simulink library "SimscapeCustomComponents_lib"  (R2025b)
settings: Solver=VariableStepAuto  StartTime=0.0  StopTime=10.0  RelTol=1e-3
undefined symbols (not defined in the file or in its folder): base, baseVdc, capacity, DiscIntNeverNeededParam, ee_sli_rtmsupport, filterInductance, freqeuncy, frequency, gcbh, gflInverter, gfmInverter, iMaxPU, Inertia, initialSOC, plantRating, solar, Ts, ups, Vac, windSystem, windTurbine
libraries: fl_lib x397, nesl_utility x171, eeGeneralControl x85, ee_lib x82, simulink x72, datacenter_lib x68, eeTransforms x38, slpidlib x24, buildingEnergy_lib x20, SimscapeFluids_lib x17, eeSinusoidalMeasurementV2 x8, eePwmGenerator x8
(part 1 of 24)
settings Model: Creator=skota  LastModifiedBy=skota

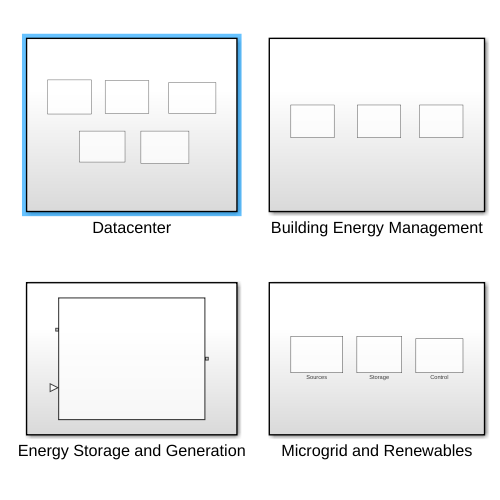
[thumbnail: Simulink's stored preview of the top-level diagram]
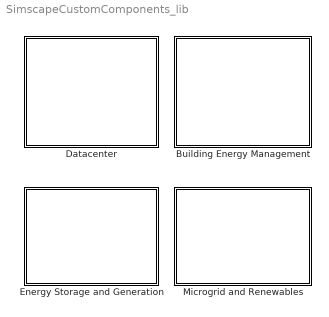
== system SimscapeCustomComponents_lib ==
  Building Energy Management : Subsystem
  Datacenter : Subsystem
  Energy Storage and Generation : Subsystem
  Microgrid and Renewables : Subsystem

== system SimscapeCustomComponents_lib/Building Energy Management ==
  Building : Subsystem
  Environment : Subsystem
  HVAC : Subsystem

== system SimscapeCustomComponents_lib/Datacenter ==
  Assemblies : Subsystem
  CDU : Subsystem
  Facilities : Subsystem
  PDU : Subsystem
  Utilities : Subsystem

== system SimscapeCustomComponents_lib/Energy Storage and Generation ==
  Vanadium Redox Flow Battery : energyStorage_lib/Vanadium Redox Flow Battery  flowrateLUT=[5, 10, 20, 40, 80] lpm  thermalManagement=vanadiumRedoxFlowThermalModel.disabled  temperatureLUT=[293, 300, 313] K  initialTsys=280 K  SOC=0.99  electrolyteDen=1000 kg/m^3  electrolyteCp=800 J/(K*kg)  electrolyteKinVis=3.9e-6 m^2/s  crossDiffModel=vanadiumRedoxFlowChemistry.disabled  thMemb=1e-3 m  diffCoeff2=4.31e-12 m^2/s  diffCoeff3=1.92e-12 m^2/s  diffCoeff4=6.53e-12 m^2/s  diffCoeff5=3.78e-12 m^2/s  activationE=17341 W*s/mol  electrolyteK=1 1/(Ohm*m)  minStateOfCharge=1e-4  maxStateOfCharge=0.9999  msgWarn=simscape.enum.assert.action.none  molar=2 mol/l  V0=1.3 V  LUTdischgR0=0.1 * ones(1, 5) Ohm  LUTdischgRes=0.1 * ones(1, 5) Ohm  LUTdischgTau=10 * ones(1, 5) s  LUTchgR0=0.1 * ones(1, 5) Ohm  LUTchgRes=0.1 * ones(1, 5) Ohm  LUTchgTau=10 * ones(1, 5) s  stackLen=0.15 m  stackWid=0.30 m  stackHgt=0.30 m  stackMassCp=324000 J/K  stackPrDropLUT=[100, 110, 120, 130, 140] Pa  pipeLength=1 m  pipeDia=1e-2 m  pipeArea=0.01 m^2  pipeRoughness=15e-6 m  Nc=20  Ns=10  Np=2  seriesFlowMalDistr=ones(1, 10)  shuntResModel=vanadiumRedoxFlowShuntCurrModel.disabled  shuntRes=1000 Ohm  containerVolume=0.5 m^3  containerArea=10 m^2  containerThermalmass=90000 J/K  nFans=5  fanCapacity=80 m^3/hr  extHTC=20 W/(K*m^2)  F=96485 C/mol  R=8.314 J/(K*mol)  Cmin=0 mol/m^3  openSw=1e-8 1/Ohm  flUnit=1 / 60000 m^3/(lpm*s)  containerAirCp=700 J/(K*kg)  containerAirDen=1.2 kg/m^3  ReLaminar=2000  ReTurbulent=4000  darcyFriction=64  vSwitchOpen_specify=off  vSwitchOpen_priority=None  vSwitchOpen=0 V  vSwitchOpen_nominal_specify=off  vSwitchOpen_nominal_value=1  vSwitchOpen_nominal_unit=V  portH_specify=off  portH_priority=None  portH=0 W  portH_nominal_specify=off  portH_nominal_value=1  portH_nominal_unit=W  tankNegT_specify=off  tankNegT_priority=High  tankNegT=298 K  tankNegT_nominal_specify=off  tankNegT_nominal_value=1  tankNegT_nominal_unit=K  tankPosT_specify=off  tankPosT_priority=High  tankPosT=298 K  tankPosT_nominal_specify=off  tankPosT_nominal_value=1  tankPosT_nominal_unit=K  i_specify=off  i_priority=None  i=0 A  i_nominal_specify=off  i_nominal_value=1  i_nominal_unit=A  is_specify=off  is_priority=None  is=0 A  is_nominal_specify=off  is_nominal_value=1  is_nominal_unit=A  systemPrDrop_specify=off  systemPrDrop_priority=None  systemPrDrop=0 Pa  systemPrDrop_nominal_specify=off  systemPrDrop_nominal_value=1  systemPrDrop_nominal_unit=Pa  shuntCurrPercent_specify=off  shuntCurrPercent_priority=None  shuntCurrPercent=0  shuntCurrPercent_nominal_specify=off  shuntCurrPercent_nominal_value=1  shuntCurrPercent_nominal_unit=1
      settings: InternalSimscapePortConfiguration="{\"Bottom\":[],\"Left\":[{\"id\":\"p\",\"label\":\"+\",\"type\":\"foundation.electrical.electrical\"},{\"id\":\"flow\",\"label\":\"lpm\",\"type\":\"input\"}],\"Right\":[{\"id\":\"n\",\"label\":\"-\",\"type\":\"foundation.electrical.electrical\"}],\"Top\":[]}"

== system SimscapeCustomComponents_lib/Microgrid and Renewables ==
  Control : Subsystem
  Sources : Subsystem
  Storage : Subsystem

== system SimscapeCustomComponents_lib/Building Energy Management/Building ==
  Room Volume : buildingEnergy_lib/Room Volume  N1=1  N2=1  iniT=300 K  length=5 m  width=3 m  height=2.5 m
      settings: InternalSimscapePortConfiguration="{\"Bottom\":[],\"Left\":[{\"id\":\"S\",\"label\":\"S\",\"type\":\"input\"}],\"Right\":[{\"id\":\"T\",\"label\":\"T\",\"type\":\"output\"}],\"Top\":[{\"id\":\"M1\",\"label\":\"M1\",\"type\":\"foundation.thermal.thermal\"},{\"id\":\"M2\",\"label\":\"M2\",\"type\":\"foundation.thermal.thermal\"}]}"
  Room Volume (HVAC) : buildingEnergy_lib/Room Volume (HVAC)  Hnum=1  length=5 m  width=3 m  height=2.5 m  airInletCrossSection=0.01 m^2  airOutletCrossSection=0.01 m^2  perPersonQ=0 W  breathT=0 K  perPersonCO2=0 g/s  perPersonMoisture=0 g/s  relHumidity=1  tauCondensation=0.001 s  entrainedFrac=1  traceGasMassFrac=0  pressureAirVol=0.101325 MPa  temperatureAirVol=293 K  relHumidityAirVol=0  mfWaterDroplets=0
      settings: InternalSimscapePortConfiguration="{\"Bottom\":[],\"Left\":[{\"id\":\"S\",\"label\":\"S\",\"type\":\"input\"},{\"id\":\"N\",\"label\":\"N\",\"type\":\"input\"},{\"id\":\"A\",\"label\":\"A\",\"type\":\"foundation.moist_air.moist_air\"}],\"Right\":[{\"id\":\"T\",\"label\":\"T\",\"type\":\"output\"},{\"id\":\"B\",\"label\":\"B\",\"type\":\"foundation.moist_air.moist_air\"}],\"Top\":[{\"id\":\"H\",\"label\":\"M\",\"type\":\"foundation.thermal.thermal\"}]}"
  Room with Air Volume : Subsystem  mask{roomWid=3, roomHgt=2.5, roomLen=5, htc=10, iniT=300, indxS=1}
      mask prompts: roomWid "Room Width (m)"; roomHgt "Room Height (m)"; roomLen "Room Length (m)"; htc "Heat Transfer Coefficient (W/K*m^2)"; iniT "Initial Temperature (K)"; indxS "Heat source vector index"
      settings: PortSchema="{\"entries\":[{\"content\":{\"sides\":[{\"content\":{\"connectorIds\":[\"LConn1\",\"LConn2\"]},\"type\":\"ConnectorPlacement.EquallySpacedRectSide\",\"uuid\":\"8440f6ae-3089-4f14-af97-f7a7d9c670fb\"},{\"content\":{\"connectorIds\":[\"RConn1\",\"RConn2\"],\"side\":\"RIGHT\"},\"type\":\"ConnectorPlacement.EquallySpacedRectSide\",\"uuid\":\"df84a625-bd6d-46a4-b71c-d411d28f8df6\"},{\"content\":{\"connectorIds\":[\"LConn3\",\"LConn4\"],\"side\":\"TOP\"},\"type\":\"ConnectorPlacement.EquallySpacedRectSide\",\"uuid\":\"90f16a0a-d00c-4f13-8e79-f2f23ea8b565\"},{\"content\":{\"connectorIds\":[\"RConn3\",\"RConn4\"],\"side\":\"BOTTOM\"},\"type\":\"ConnectorPlacement.EquallySpacedRectSide\",\"uuid\":\"4eb9d9d9-e9b4-43a3-a1e1-726815f3b9ff\"}]},\"type\":\"ConnectorPlacement.EquallySpacedConnector\",\"uuid\":\"51dc529f-94b8-407e-b287-301b2c0c8383\"}],\"packageUris\":[\"http://schema.mathworks.com/mf0/Connector/R2020b\"],\"version\":\"1.0\"}"
      mask Help: web("DocumentationCompositeRoom.html")
      mask DialogControl DescGroupVar Prompt: Description
      mask DialogControl DescTextVar Prompt: Room model with air volume.
      mask DialogControl ParameterGroupRoom Prompt: Room Dimensions
      mask DialogControl ParameterGroupHT Prompt: Heat Transfer
      mask Display: image("roomWithAirVolume.png");
  Room with Radiator : Subsystem  mask{pipeRoughnessR=1e-6, pipeLenR=10, pipeCrossSectionalAreaR=1.75e-4, pipeHydrDiaR=1.5e-2, roomWid=3, roomHgt=2.5, roomLen=5, htc=10, iniT=300, indxS=1, indxV=1}
      mask prompts: pipeRoughnessR "Pipe roughness (m)"; pipeLenR "Pipe length (m)"; pipeCrossSectionalAreaR "Pipe cross-sectional area (m^2)"; pipeHydrDiaR "Pipe hydraulic diameter (m)"; roomWid "Room Width (m)"; roomHgt "Room Height (m)"; roomLen "Room Length (m)"; htc "Heat Transfer Coefficient (W/K*m^2)"; iniT "Initial Temperature (K)"; indxS "Heat source vector index"; indxV "Valve operation vector index"
      settings: PortSchema="{\"entries\":[{\"content\":{\"sides\":[{\"content\":{\"connectorIds\":[\"LConn1\",\"LConn2\",\"LConn3\",\"LConn4\"]},\"type\":\"ConnectorPlacement.EquallySpacedRectSide\",\"uuid\":\"8440f6ae-3089-4f14-af97-f7a7d9c670fb\"},{\"content\":{\"connectorIds\":[\"RConn1\",\"RConn2\",\"RConn3\"],\"side\":\"RIGHT\"},\"type\":\"ConnectorPlacement.EquallySpacedRectSide\",\"uuid\":\"df84a625-bd6d-46a4-b71c-d411d28f8df6\"},{\"content\":{\"connectorIds\":[\"LConn5\",\"LConn6\"],\"side\":\"TOP\"},\"type\":\"ConnectorPlacement.EquallySpacedRectSide\",\"uuid\":\"90f16a0a-d00c-4f13-8e79-f2f23ea8b565\"},{\"content\":{\"connectorIds\":[\"RConn4\",\"RConn5\"],\"side\":\"BOTTOM\"},\"type\":\"ConnectorPlacement.EquallySpacedRectSide\",\"uuid\":\"4eb9d9d9-e9b4-43a3-a1e1-726815f3b9ff\"}]},\"type\":\"ConnectorPlacement.EquallySpacedConnector\",\"uuid\":\"51dc529f-94b8-407e-b287-301b2c0c8383\"}],\"packageUris\":[\"http://schema.mathworks.com/mf0/Connector/R2020b\"],\"version\":\"1.0\"}"
      mask Help: web("DocumentationCompositeRoomRadiator.html")
      mask DialogControl DescGroupVar Prompt: Description
      mask DialogControl DescTextVar Prompt: Room model with radiator for thermal comfort.
      mask DialogControl ParameterGroupRadiator Prompt: Radiator
      mask DialogControl ParameterGroupRoom Prompt: Room Dimensions
      mask DialogControl ParameterGroupHT Prompt: Heat Transfer
      mask Display: image("roomWithRadiator.png");
  Room with Under-floor Piping : Subsystem  mask{pipeRoughnessUFP=1e-6, pipeLenUFP=50, pipeCrossSectionalAreaUFP=1.75e-4, pipeHydrDiaUFP=1.5e-2, thermalResFloor=100, roomWid=3, roomHgt=2.5, roomLen=5, htc=10, iniT=300, indxS=1, indxV=1}
      mask prompts: pipeRoughnessUFP "Pipe roughness (m)"; pipeLenUFP "Pipe length (m)"; pipeCrossSectionalAreaUFP "Pipe cross-sectional area (m^2)"; pipeHydrDiaUFP "Pipe hydraulic diameter (m)"; thermalResFloor "Thermal resistance to floor (K/W)"; roomWid "Room Width (m)"; roomHgt "Room Height (m)"; roomLen "Room Length (m)"; htc "Heat Transfer Coefficient (W/K*m^2)"; iniT "Initial Temperature (K)"; indxS "Heat source vector index"; indxV "Valve operation vector index"
      settings: PortSchema="{\"entries\":[{\"content\":{\"sides\":[{\"content\":{\"connectorIds\":[\"LConn1\",\"LConn2\",\"LConn3\",\"LConn4\"]},\"type\":\"ConnectorPlacement.EquallySpacedRectSide\",\"uuid\":\"8440f6ae-3089-4f14-af97-f7a7d9c670fb\"},{\"content\":{\"connectorIds\":[\"RConn1\",\"RConn2\",\"RConn3\"],\"side\":\"RIGHT\"},\"type\":\"ConnectorPlacement.EquallySpacedRectSide\",\"uuid\":\"df84a625-bd6d-46a4-b71c-d411d28f8df6\"},{\"content\":{\"connectorIds\":[\"LConn5\",\"LConn6\"],\"side\":\"TOP\"},\"type\":\"ConnectorPlacement.EquallySpacedRectSide\",\"uuid\":\"90f16a0a-d00c-4f13-8e79-f2f23ea8b565\"},{\"content\":{\"connectorIds\":[\"RConn4\",\"RConn5\"],\"side\":\"BOTTOM\"},\"type\":\"ConnectorPlacement.EquallySpacedRectSide\",\"uuid\":\"4eb9d9d9-e9b4-43a3-a1e1-726815f3b9ff\"}]},\"type\":\"ConnectorPlacement.EquallySpacedConnector\",\"uuid\":\"51dc529f-94b8-407e-b287-301b2c0c8383\"}],\"packageUris\":[\"http://schema.mathworks.com/mf0/Connector/R2020b\"],\"version\":\"1.0\"}"
      mask Help: web("DocumentationCompositeRoomUFP.html")
      mask DialogControl DescGroupVar Prompt: Description
      mask DialogControl DescTextVar Prompt: Room model with under-floor piping for thermal comfort.
      mask DialogControl ParameterGroupUFP Prompt: Under Floor Piping
      mask DialogControl ParameterGroupRoom Prompt: Room Dimensions
      mask DialogControl ParameterGroupHT Prompt: Heat Transfer
      mask Display: image("roomWithUFP.png");
  "Room, Radiator, and Under-floor Piping" : Subsystem  mask{pipeRoughnessR=1e-6, pipeLenR=10, pipeCrossSectionalAreaR=1.75e-4, pipeHydrDiaR=1.5e-2, pipeRoughnessUFP=1e-6, pipeLenUFP=50, pipeCrossSectionalAreaUFP=1.75e-4, pipeHydrDiaUFP=1.5e-2, thermalResFloor=100, roomWid=3, roomHgt=2.5, roomLen=5, htc=10, iniT=300, indxS=1, indxV=1}
      mask prompts: pipeRoughnessR "Pipe roughness (m)"; pipeLenR "Pipe length (m)"; pipeCrossSectionalAreaR "Pipe cross-sectional area (m^2)"; pipeHydrDiaR "Pipe hydraulic diameter (m)"; pipeRoughnessUFP "Pipe roughness (m)"; pipeLenUFP "Pipe length (m)"; pipeCrossSectionalAreaUFP "Pipe cross-sectional area (m^2)"; pipeHydrDiaUFP "Pipe hydraulic diameter (m)"; thermalResFloor "Thermal resistance to floor (K/W)"; roomWid "Room Width (m)"; roomHgt "Room Height (m)"; roomLen "Room Length (m)"; htc "Heat Transfer Coefficient (W/K*m^2)"; iniT "Initial Temperature (K)"; indxS "Heat source vector index"; indxV "Valve operation vector index"
      settings: PortSchema="{\"entries\":[{\"content\":{\"sides\":[{\"content\":{\"connectorIds\":[\"LConn1\",\"LConn2\",\"LConn3\",\"LConn4\"]},\"type\":\"ConnectorPlacement.EquallySpacedRectSide\",\"uuid\":\"8440f6ae-3089-4f14-af97-f7a7d9c670fb\"},{\"content\":{\"connectorIds\":[\"RConn1\",\"RConn2\",\"RConn3\"],\"side\":\"RIGHT\"},\"type\":\"ConnectorPlacement.EquallySpacedRectSide\",\"uuid\":\"df84a625-bd6d-46a4-b71c-d411d28f8df6\"},{\"content\":{\"connectorIds\":[\"LConn5\",\"LConn6\"],\"side\":\"TOP\"},\"type\":\"ConnectorPlacement.EquallySpacedRectSide\",\"uuid\":\"90f16a0a-d00c-4f13-8e79-f2f23ea8b565\"},{\"content\":{\"connectorIds\":[\"RConn4\",\"RConn5\"],\"side\":\"BOTTOM\"},\"type\":\"ConnectorPlacement.EquallySpacedRectSide\",\"uuid\":\"4eb9d9d9-e9b4-43a3-a1e1-726815f3b9ff\"}]},\"type\":\"ConnectorPlacement.EquallySpacedConnector\",\"uuid\":\"51dc529f-94b8-407e-b287-301b2c0c8383\"}],\"packageUris\":[\"http://schema.mathworks.com/mf0/Connector/R2020b\"],\"version\":\"1.0\"}"
      mask Help: web("DocumentationCompositeRoomRadiatorUFP.html")
      mask DialogControl DescGroupVar Prompt: Description
      mask DialogControl DescTextVar Prompt: Room model with radiator and under-floor piping for thermal comfort.
      mask DialogControl ParameterGroupRadiator Prompt: Radiator
      mask DialogControl ParameterGroupUFP Prompt: Under Floor Piping
      mask DialogControl ParameterGroupRoom Prompt: Room Dimensions
      mask DialogControl ParameterGroupHT Prompt: Heat Transfer
      mask Display: image("roomWithRadiatorAndUFP.png");
  Wall External : buildingEnergy_lib/Wall External  extWallModel=wallExternalModelOption.wallSolarWinVent  wallLength=5 m  wallHeight=3 m  wallThickness=0.3 m  wallMaterialDen=4000 kg/m^3  wallMaterialCp=1870 J/(K*kg)  wallAbsorptivity=0.5  wallThermalK=2 W/(K*m)  winLength=1 m  winHeight=0.5 m  winThickness=0.007 m  winMaterialDen=2500 kg/m^3  winMaterialCp=787 J/(K*kg)  winAbsorptivity=0.35  winThermalK=1 W/(K*m)  winTransmissivity=0.45  ventLength=0.1 m  ventHeight=0.1 m  extToWallHTC=5 W/(K*m^2)  intToRoomHTC=5 W/(K*m^2)  iniT=300 K  latitude=5  longitude=5  localTime=5  dayLightS=0  surfAngle=90 deg  surfUnitV=[0, -1]  startYear=2025  startMonth=1  startDay=1  startHr=1  numHrsData=24  interp_method=simscape.enum.interpolation.linear  extrap_method=simscape.enum.extrapolation.nearest
      settings: InternalSimscapePortConfiguration="{\"Bottom\":[],\"Left\":[{\"id\":\"R\",\"label\":\"Rad\",\"type\":\"input\"},{\"id\":\"A\",\"label\":\"A\",\"type\":\"foundation.thermal.thermal\"}],\"Right\":[{\"id\":\"B\",\"label\":\"B\",\"type\":\"foundation.thermal.thermal\"}],\"Top\":[]}"
  Wall Selector : buildingEnergy_lib/Wall Selector  optWall=wallModelOption.wallSolarWinVent  wallLength=5 m  wallHeight=3 m  wallThickness=0.3 m  wallMaterialDen=4000 kg/m^3  wallMaterialCp=1870 J/(K*kg)  wallAbsorptivity=0.5  wallThermalK=2 W/(K*m)  winLength=1 m  winHeight=0.5 m  winThickness=0.007 m  winMaterialDen=2500 kg/m^3  winMaterialCp=787 J/(K*kg)  winAbsorptivity=0.35  winThermalK=1 W/(K*m)  winTransmissivity=0.45  ventLength=0.1 m  ventHeight=0.1 m  extToWallHTC=5 W/(K*m^2)  intToRoomHTC=5 W/(K*m^2)  iniT=300 K
      settings: InternalSimscapePortConfiguration="{\"Bottom\":[],\"Left\":[{\"id\":\"S\",\"label\":\"S\",\"type\":\"input\"},{\"id\":\"A\",\"label\":\"A\",\"type\":\"foundation.thermal.thermal\"}],\"Right\":[{\"id\":\"B\",\"label\":\"B\",\"type\":\"foundation.thermal.thermal\"}],\"Top\":[]}"

== system SimscapeCustomComponents_lib/Building Energy Management/Environment ==
  Day Scheduler : buildingEnergy_lib/Day Scheduler  numRoom=30  roomIndex=[1 : 30]  heatSource=ones(30, 24) W  t=1 : 24  oneHr=3600
      settings: InternalSimscapePortConfiguration="{\"Bottom\":[],\"Left\":[],\"Right\":[{\"id\":\"S\",\"label\":\"S\",\"type\":\"output\"}],\"Top\":[]}"
  Solar Radiation (LUT) : buildingEnergy_lib/Solar Radiation (LUT)  latitude=5  longitude=5  localTime=5  dayLightS=0  startYear=2025  startMonth=1  startDay=1  startHr=1  numHrsData=24  cloudData=cloudCoverLibOption.none  cloudCoverVal=zeros(1, 24)  interp_method=simscape.enum.interpolation.linear  extrap_method=simscape.enum.extrapolation.nearest
      settings: InternalSimscapePortConfiguration="{\"Bottom\":[],\"Left\":[],\"Right\":[{\"id\":\"S\",\"label\":\"Rad\",\"type\":\"output\"}],\"Top\":[]}"
  Solar Radiation On Surface : buildingEnergy_lib/Solar Radiation On Surface  latitude=5  longitude=5  localTime=5  dayLightS=0  surfAngle=90 deg  surfUnitV=[0, -1]  startYear=2025  startMonth=1  startDay=1  startHr=1  numHrsData=24  interp_method=simscape.enum.interpolation.linear  extrap_method=simscape.enum.extrapolation.nearest
      settings: InternalSimscapePortConfiguration="{\"Bottom\":[],\"Left\":[{\"id\":\"S\",\"label\":\"Rad\",\"type\":\"input\"}],\"Right\":[{\"id\":\"Sf\",\"label\":\"S\",\"type\":\"output\"}],\"Top\":[]}"
  Temperature Source (LUT) : buildingEnergy_lib/Temperature Source (LUT)  latitude=5  longitude=5  localTime=5  dayLightS=0  startYear=2025  startMonth=1  startDay=1  startHr=1  numDaysData=10  interp_method=simscape.enum.interpolation.linear  extrap_method=simscape.enum.extrapolation.error  avgDayTvec=300 * ones(1, 10) K  pcDayTvar=5  avgNightTvec=300 * ones(1, 10) K  pcNightTvar=5
      settings: InternalSimscapePortConfiguration="{\"Bottom\":[],\"Left\":[],\"Right\":[{\"id\":\"H\",\"label\":\"H\",\"type\":\"foundation.thermal.thermal\"}],\"Top\":[]}"

== system SimscapeCustomComponents_lib/Building Energy Management/HVAC ==
  Air Water Heat Pump : buildingEnergy_lib/Air Water Heat Pump  nominalCapacityA=200 kW  seasonalCOPvalA=3.1  nominalCapacityB=200 kW  seasonalCOPvalB=3.1  nominalCapacityC=200 kW  seasonalCOPvalC=3.1  nominalCapacityD=200 kW  seasonalCOPvalD=3.1  nominalCapacityE=200 kW  seasonalCOPvalE=3.1  nominalCapacityF=200 kW  seasonalCOPvalF=3.1  backupElecHeater=0 kW  wInletOpRangeUpp=330 K  wInletOpRangeLow=278 K  airTemperatureVector=273 + [-2, -2, 7, 7, 35, 35]  waterTemperatureVector=273 + [55, 65, 35, 45, 18, 7]  waterSpHeat=4186 J/(K*kg)  smallPower=1e-3 W  maxCOP_specify=off  maxCOP_priority=None  maxCOP=8  maxCOP_nominal_specify=off  maxCOP_nominal_value=1  maxCOP_nominal_unit=1
      settings: InternalSimscapePortConfiguration="{\"Bottom\":[{\"id\":\"Ta\",\"label\":\"Ta\",\"type\":\"input\"},{\"id\":\"Tw\",\"label\":\"Tw\",\"type\":\"input\"}],\"Left\":[{\"id\":\"Tl\",\"label\":\"Tl\",\"type\":\"input\"},{\"id\":\"Fw\",\"label\":\"Fw\",\"type\":\"input\"},{\"id\":\"Op\",\"label\":\"Op\",\"type\":\"input\"},{\"id\":\"Ep\",\"label\":\"Ep\",\"type\":\"input\"},{\"id\":\"Nd\",\"label\":\"Nd\",\"type\":\"input\"}],\"Right\":[{\"id\":\"calcCap\",\"label\":\"Q\",\"type\":\"output\"},{\"id\":\"calcCOP\",\"label\":\"COP\",\"type\":\"output\"},{\"id\":\"ePower\",\"label\":\"ePow\",\"type\":\"output\"}],\"Top\":[]}"
  Air Water Heat Pump (TL) : Subsystem  mask{heatingCapacityA=10.17, heatingCoPA=4.86, heatingCapacityB=10.12, heatingCoPB=3.7, heatingCapacityC=10.17, heatingCoPC=4.86, heatingCapacityD=10.12, heatingCoPD=3.7, coolingCapacityE=10.55, coolingCoPE=4.13, coolingCapacityF=6.9, coolingCoPF=2.7, elecHeaterPower=0, coilLen=2, coilArea=pi*(5e-2^2)/4, coilDia=5e-2, tankVolume=5, initialT=299.8, waterOpTempMax=330, waterOpTempMin=278, initialP=0.101325, measTimelagWater=60, minWaterFlowRate=1e-3, nomFlowDuringTest=0.5}
      mask prompts: heatingCapacityA "A-2W55, estimated heating capacity (kW)"; heatingCoPA "A-2W55, estimated COP (or SCOP)"; heatingCapacityB "A-2W65, estimated heating capacity (kW)"; heatingCoPB "A-2W65, estimated COP (or SCOP)"; heatingCapacityC "A7W35, estimated heating capacity (kW)"; heatingCoPC "A7W35, estimated COP (or SCOP)"; heatingCapacityD "A7W45, estimated heating capacity (kW)"; heatingCoPD "A7W45, estimated COP (or SCOP)"; coolingCapacityE "A35W18, estimated cooling capacity (kW)"; coolingCoPE "A35W18, estimated COP (or SCOP)"; coolingCapacityF "A35W7, estimated cooling capacity (kW)"; coolingCoPF "A35W7, estimated COP (or SCOP)"; elecHeaterPower "Additional electric heater rating (kW)"; coilLen "Length of coil pipe (m)"; coilArea "Area of coil pipe (m^2)"; coilDia "Diameter of coil pipe (m)"; tankVolume "Heat exchanger internal volume (m^3)"; initialT "Initial Temperature (K)"; waterOpTempMax "Maximum operational water temperature"; waterOpTempMin "Minimum operation water temperature"; initialP "Initial pressure of coil pipe water (MPa)"; measTimelagWater "Temperature sensor delay for water flow (s)"; minWaterFlowRate "Minimum water flowrate (kg/s)"; nomFlowDuringTest "Nominal water flowrate during test (kg/s)"
      mask Help: web("DocumentationAirWaterHeatPumpTL.html")
      mask DialogControl DescGroupVar Prompt: Description
      mask DialogControl DescTextVar Prompt: Heat pump model based on EN14511 test data.
      mask DialogControl Container3 Prompt: EN14511 (Heating) Data
      mask DialogControl Container4 Prompt: EN14511 (Cooling) Data
      mask DialogControl ParameterGroupVar Prompt: Heat Pump Construction
      mask DialogControl Container5 Prompt: Flow and Thermal Specifications
      mask Display: image('AirWaterHeatPumpTL.png');
  Heat Source Control : Subsystem  mask{capacity=12000, num=1, delT=10, tau=1, iniT=280}
      mask prompts: capacity "Heat pump capacity (W)"; num "Number of sources (-)"; delT "Change in water temperature (deg C)"; tau "Measurement time constant (s)"; iniT "Initial water temperature (K)"
      mask Help: web("DocumentationCompositeHeatSourceControl.html")
      mask DialogControl DescGroupVar Prompt: Description
      mask DialogControl DescTextVar Prompt: The block evaluates heating or cooling requirements for a building  based on the measured room temperatures and the specified set point temperature.
      mask DialogControl HeatPump Prompt: Heat Pump
      mask Display: image('HeatSourceControlIcon.png');
  Room Underfloor Piping : buildingEnergy_lib/Room Underfloor Piping  pipeHydrDia=1.5e-2 m  pipeLength=1 m  pipeArea=1.75e-4 m^2  pipeRoughness=1e-6 m  htc=10 W/(K*m^2)  iniTemperature=300 K
      settings: InternalSimscapePortConfiguration="{\"Bottom\":[],\"Left\":[{\"id\":\"TL_V\",\"label\":\"V\",\"type\":\"input\"},{\"id\":\"TL_A\",\"label\":\"A\",\"type\":\"foundation.thermal_liquid.thermal_liquid\"}],\"Right\":[{\"id\":\"M\",\"label\":\"R\",\"type\":\"foundation.thermal.thermal\"},{\"id\":\"TL_B\",\"label\":\"B\",\"type\":\"foundation.thermal_liquid.thermal_liquid\"}],\"Top\":[]}"
  Room Wall Radiator : buildingEnergy_lib/Room Wall Radiator  pipeHydrDia=1.5e-2 m  pipeLength=1 m  pipeArea=1.75e-4 m^2  pipeRoughness=1e-6 m  htc=10 W/(K*m^2)  iniTemperature=300 K
      settings: InternalSimscapePortConfiguration="{\"Bottom\":[],\"Left\":[{\"id\":\"TL_V\",\"label\":\"V\",\"type\":\"input\"},{\"id\":\"TL_A\",\"label\":\"A\",\"type\":\"foundation.thermal_liquid.thermal_liquid\"}],\"Right\":[{\"id\":\"M\",\"label\":\"R\",\"type\":\"foundation.thermal.thermal\"},{\"id\":\"TL_B\",\"label\":\"B\",\"type\":\"foundation.thermal_liquid.thermal_liquid\"}],\"Top\":[]}"

== system SimscapeCustomComponents_lib/Datacenter/Assemblies ==
  Air Cooled PDU Assembly : Subsystem  mask{nAssembly=3, nRacks=4, nTrays=6, nFans=5, flowVec=[0.1 0.2 0.3 0.4 0.5], prDropVec=[50 100 150 220 280], fanEffVec=[0.58, 0.60, 0.61, 0.60, 0.59], trayMass=5, trayCp=2000, trayThermalR=0.1, nGPU=1, gpuTDPperDie=1200, gpuIdlePower=300, gpuHBMpower=80, gpuExponent=1.4, gpuHBMutil=0.7, gpuLeakage=1.5, gpuNominalDieT=350, gpuDieThermalC=50, gpuHeatSinkR=0.15, gpuSurfArea=0.01, gpuAmbientR=0.5, nCPU=1, cpuTDPperSocket=350, cpuIdlePower=80, cpuExponent=1.1, cpuLeakage=1.5, cpuNominalDieT=350, cpuDieThermalC=50, cpuHeatSinkR=0.15, cpuSurfArea=0.01, cpuAmbientR=0.5, initialT=350, htc=10}
      mask prompts: nAssembly "Number of PDU + Fan assemblies (-)"; nRacks "Number of racks per PDU (-)"; nTrays "Number of IT trays per rack (-)"; nFans "Number of fans per assembly (-)"; flowVec "Fan flow rate vector (m^3/s)"; prDropVec "Fan pressure drop vector (Pa)"; fanEffVec "Fan efficiency vector, 0-1 (-)"; trayMass "Tray mass (kg)"; trayCp "Tray specific heat capacity (J/kg*K)"; trayThermalR "Tray to external thermal resistance (K/W)"; nGPU "Number of GPU per tray (-)"; gpuTDPperDie "GPU TDP per die (W)"; gpuIdlePower "GPU idle power (W)"; gpuHBMpower "HBM power per GPU (W)"; gpuExponent "GPU power utilization exponent (-)"; gpuHBMutil "HBM utilization as fraction of compute utilization (-)"; gpuLeakage "Leakage increase per K above nominal temperature (W/K)"; gpuNominalDieT "Nominal die temperature at TDP (K)"; gpuDieThermalC "GPU die thermal capacitance (J/K)"; gpuHeatSinkR "GPU die-heat-sink thermal resistance (K/W)"; gpuSurfArea "Surface area per die for ambient heat transfer (m^2)"; gpuAmbientR "GPU die-ambient thermal resistance (K/W)"; nCPU "Number of CPU per tray (-)"; cpuTDPperSocket "CPU TDP per socket (W)"; cpuIdlePower "CPU idle power per socket (W)"; cpuExponent "CPU power utilization exponent (-)"; cpuLeakage "Leakage increase per K above nominal temperature (W/K)"; cpuNominalDieT "Nominal die temperature at TDP (K)"; cpuDieThermalC "CPU die thermal capacitance (J/K)"; cpuHeatSinkR "CPU die-heat-sink thermal resistance (K/W)"; cpuSurfArea "Surface area per die for ambient heat transfer (m^2)"; cpuAmbientR "CPU die-ambient thermal resistance (K/W)"; initialT "Initial temperature (K)"; htc "Heat transfer coefficient to ambient (W/m^2.K)"
      settings: CopyFcn=set_param(gcbh,'LinkStatus','none');
      mask Help: web("DocumentationAirCooledPDUAssembly.html")
      mask DialogControl Container10 Prompt: PDU Racks
      mask DialogControl getRatingButton Prompt: Get Rating
      mask DialogControl Container11 Prompt: Fans
      mask DialogControl Container9 Prompt: IT Tray
      mask DialogControl Container6 Prompt: GPU
      mask DialogControl Container7 Prompt: CPU
      mask DialogControl Container8 Prompt: Initial Conditions
      mask Display: image('icon_AssemblyAirCooled.png');
  PDU + CDU Assembly (LUT) : Subsystem  mask{nAssembly=3, nRacks=3, nTrays=6, flowrate_vec=[0.3, 0.5, 1.0, 1.3, 1.7, 2, 2.6, 3.3, 3.5, 3.7]/998, capacity_vec=50000*[0.32, 0.35, 0.40, 0.42, 0.43, 0.43, 0.44, 0.45, 0.46, 0.47], numPump=2, effPump_vec=[0.4,0.42,0.45,0.5,0.55,0.6,0.62,0.65,0.65,0.64], prDrop_mat=100000*[0.28,1.11,2.5,4.44,6.94,10,13.61,17.78,22.5,27.78; 5.6,2.22,5,8.88,13.88,20,27.22,35.56,45,55.56]', speed=2, trayMass=5, trayCp=2000, trayThermalR=0.1, nGPU=1, gpuTDPperDie=1200, gpuIdlePower=300, gpuHBMpower=80, gpuExponent=1.4, gpuHBMutil=0.7, gpuLeakage=1.5, gpuNominalDieT=350, gpuDieThermalC=50, gpuHeatSinkR=0.15, gpuSurfArea=0.01, gpuAmbientR=0.5, nCPU=1, cpuTDPperSocket=350, cpuIdlePower=80, cpuExponent=1.1, cpuLeakage=1.5, cpuNominalDieT=350, cpuDieThermalC=50, cpuHeatSinkR=0.15, cpuSurfArea=0.01, cpuAmbientR=0.5, initialT=350, htc=10}
      mask prompts: nAssembly "Number of PDU+CDU assemblies (-)"; nRacks "Number of racks (-)"; nTrays "Number of IT trays per rack (-)"; flowrate_vec "Coolant volumetric flowrate vector (m^3/s)"; capacity_vec "Heat exchanger capacity vector (W)"; numPump "Total number of pumps in each assembly (-)"; effPump_vec "Pump efficiency vector, 0-1 (-)"; prDrop_mat "Pressure drop (Pa)"; speed "Pump speed scaling (-)"; trayMass "Tray mass (kg)"; trayCp "Tray specific heat capacity (J/kg*K)"; trayThermalR "Tray to external thermal resistance (K/W)"; nGPU "Number of GPU per tray (-)"; gpuTDPperDie "GPU TDP per die (W)"; gpuIdlePower "GPU idle power (W)"; gpuHBMpower "HBM power per GPU (W)"; gpuExponent "GPU power utilization exponent (-)"; gpuHBMutil "HBM utilization as fraction of compute utilization (-)"; gpuLeakage "Leakage increase per K above nominal temperature (W/K)"; gpuNominalDieT "Nominal die temperature at TDP (K)"; gpuDieThermalC "GPU die thermal capacitance (J/K)"; gpuHeatSinkR "GPU die-heat-sink thermal resistance (K/W)"; gpuSurfArea "Surface area per die for ambient heat transfer (m^2)"; gpuAmbientR "GPU die-ambient thermal resistance (K/W)"; nCPU "Number of CPU per tray (-)"; cpuTDPperSocket "CPU TDP per socket (W)"; cpuIdlePower "CPU idle power per socket (W)"; cpuExponent "CPU power utilization exponent (-)"; cpuLeakage "Leakage increase per K above nominal temperature (W/K)"; cpuNominalDieT "Nominal die temperature at TDP (K)"; cpuDieThermalC "CPU die thermal capacitance (J/K)"; cpuHeatSinkR "CPU die-heat-sink thermal resistance (K/W)"; cpuSurfArea "Surface area per die for ambient heat transfer (m^2)"; cpuAmbientR "CPU die-ambient thermal resistance (K/W)"; initialT "Initial temperature (K)"; htc "Heat transfer coefficient to ambient (W/m^2.K)"
      settings: CopyFcn=set_param(gcbh,'LinkStatus','none');
      mask Help: web("DocumentationPDUCDUAssemblyLUT.html")
      mask DialogControl Container10 Prompt: PDU Racks
      mask DialogControl getRatingButton Prompt: Get Rating
      mask DialogControl Container11 Prompt: CDU
      mask DialogControl Container9 Prompt: IT Tray
      mask DialogControl Container6 Prompt: GPU
      mask DialogControl Container7 Prompt: CPU
      mask DialogControl Container8 Prompt: Initial Conditions
      mask Display: image('icon_AssemblyLUT.png');
  PDU + CDU Assembly (TL) : Subsystem  mask{nAssembly=3, nTrays=6, nRacks=4, nPumps=1, pumpNominalRPM=3500, pumpCapacityVec=2:2:24, pumpRefHeadVec=[239, 238.5, 232, 230, 222, 216, 208, 196, 186, 170,150,130], pumpRefBrkPowVec=[0.3,0.4,0.45,0.5,0.55,0.6,0.65,0.7,0.75,0.78,0.79,0.798], pumpEff=[20,40,50,60,65,70,75,75,75,73,68,60]/100, speedLimFactor=1, pumpImpellerDiaFactor=1, extFluidMdot=[.3, .5, 1, 1.3, 1.7, 2, 2.6, 3.3], extFluidPrDrop=ones(1,8), extFluidVol=0.01, extFluidPipeArea=0.01, intFluidMdot=[.3, .5, .6, .7, 1, 1.4, 1.9, 2.3], intFluidPrDrop=ones(1,8), intFluidVol=0.01, intFluidPipeArea=0.01, spDissipationTbl=[.324, .3533, .404, .4253, .4333, .4373, .4453, .4533; .3813, .424, .496, .5307, .544, .5547, .5693, .5787; .4267, .4827, .5813, .6173, .6413, .6573, .672, .6827; .4613, .528, .64, .6987, .7267, .7467, .7707, .7853; .5533, .6467, .8227, .928, .9853, 1.0187, 1.0653, 1.0973; .58, .688, .8853, 1.0147, 1.08, 1.124, 1.176, 1.2147; .624, .7467, .992, 1.148, 1.244, 1.304, 1.3773, 1.4267; .656, .7907, 1.0667, 1.26, 1.376, 1.452, 1.548, 1.612], effPipeLen=5, refT=293, refP=0.101325, refDensity=998, trayMass=5, trayCp=2000, trayThermalR=0.1, nGPU=1, gpuTDPperDie=1200, gpuIdlePower=300, gpuHBMpower=80, gpuExponent=1.4, gpuHBMutil=0.7, gpuLeakage=1.5, gpuNominalDieT=350, gpuDieThermalC=50, gpuHeatSinkR=0.15, gpuSurfArea=0.01, gpuAmbientR=0.5, nCPU=1, cpuTDPperSocket=350, cpuIdlePower=80, cpuExponent=1.1, cpuLeakage=1.5, cpuNominalDieT=350, cpuDieThermalC=50, cpuHeatSinkR=0.15, cpuSurfArea=0.01, cpuAmbientR=0.5, initialT=350, initialP=0.101325, htc=10}
      mask prompts: nAssembly "Number of PDU+CDU assemblies (-)"; nTrays "Number of IT trays per rack (-)"; nRacks "Number of racks (-)"; nPumps "Total number of pumps (-)"; pumpNominalRPM "Pump nominal rating (rpm)"; pumpCapacityVec "Reference capacity vector for each pump (m^3/s)"; pumpRefHeadVec "Reference head vector for each pump (m)"; pumpRefBrkPowVec "Reference brake power vector (kW)"; pumpEff "Electrical efficiency vector, 0-1 (-)"; speedLimFactor "Pump speed upper limit factor (-)"; pumpImpellerDiaFactor "Impeller diameter scale factor (-)"; extFluidMdot "External liquid loop mass flow rate vector (kg/s)"; extFluidPrDrop "External liquid loop pressure drop vector (kPa)"; extFluidVol "External liquid volume in heat exchanger (m^3)"; extFluidPipeArea "External liquid loop pipe cross-sectional area (m^2)"; intFluidMdot "Internal liquid loop mass flow rate vector (kg/s)"; intFluidPrDrop "Internal liquid loop pressure drop vector (kPa)"; intFluidVol "Internal liquid volume in heat exchanger (m^3)"; intFluidPipeArea "Internal liquid loop pipe cross-sectional area (m^2)"; spDissipationTbl "Specific dissipation table, SD[mdot_int,mdot_ext] (kW/K)"; effPipeLen "Effective pipe length for rack cooling (m)"; refT "Reference flow temperature (K)"; refP "Reference flow pressure (MPa)"; refDensity "Reference density for internal liquid (kg/m^3)"; trayMass "Tray mass (kg)"; trayCp "Tray specific heat capacity (J/kg*K)"; trayThermalR "Tray to external thermal resistance (K/W)"; nGPU "Number of GPU per tray (-)"; gpuTDPperDie "GPU TDP per die (W)"; gpuIdlePower "GPU idle power (W)"; gpuHBMpower "HBM power per GPU (W)"; gpuExponent "GPU power utilization exponent (-)"; gpuHBMutil "HBM utilization as fraction of compute utilization (-)"; gpuLeakage "Leakage increase per K above nominal temperature (W/K)"; gpuNominalDieT "Nominal die temperature at TDP (K)"; gpuDieThermalC "GPU die thermal capacitance (J/K)"; gpuHeatSinkR "GPU die-heat-sink thermal resistance (K/W)"; gpuSurfArea "Surface area per die for ambient heat transfer (m^2)"; gpuAmbientR "GPU die-ambient thermal resistance (K/W)"; nCPU "Number of CPU per tray (-)"; cpuTDPperSocket "CPU TDP per socket (W)"; cpuIdlePower "CPU idle power per socket (W)"; cpuExponent "CPU power utilization exponent (-)"; cpuLeakage "Leakage increase per K above nominal temperature (W/K)"; cpuNominalDieT "Nominal die temperature at TDP (K)"; cpuDieThermalC "CPU die thermal capacitance (J/K)"; cpuHeatSinkR "CPU die-heat-sink thermal resistance (K/W)"; cpuSurfArea "Surface area per die for ambient heat transfer (m^2)"; cpuAmbientR "CPU die-ambient thermal resistance (K/W)"; initialT "Initial temperature (K)"; initialP "Initial pressure (MPa)"; htc "Heat transfer coefficient to ambient (W/m^2.K)"
      settings: CopyFcn=set_param(gcbh,'LinkStatus','none');  PortSchema="{\"entries\":[{\"content\":{\"sides\":[{\"content\":{\"connectorIds\":[\"LConn1\",\"LConn2\",\"LConn3\",\"LConn4\",\"LConn5\"]},\"type\":\"ConnectorPlacement.EquallySpacedRectSide\",\"uuid\":\"c3c2deed-cbbd-4247-9ad8-92266cae4888\"},{\"content\":{\"connectorIds\":[\"RConn1\",\"RConn2\",\"RConn3\",\"RConn4\"],\"side\":\"RIGHT\"},\"type\":\"ConnectorPlacement.EquallySpacedRectSide\",\"uuid\":\"76c347ba-a09e-43ac-9cd7-77a64cbfa06b\"},{\"content\":{\"side\":\"TOP\"},\"type\":\"ConnectorPlacement.EquallySpacedRectSide\",\"uuid\":\"42a451f0-8c6e-4292-b7e5-775225f62bd3\"},{\"content\":{\"connectorIds\":[\"RConn5\",\"RConn6\"],\"side\":\"BOTTOM\"},\"type\":\"ConnectorPlacement.EquallySpacedRectSide\",\"uuid\":\"cd4c05de-d563-4aeb-b6ce-436a52495d26\"}]},\"type\":\"ConnectorPlacement.EquallySpacedConnector\",\"uuid\":\"03434805-a51b-483c-9948-e3fbab74b7d0\"}],\"packageUris\":[\"http://schema.mathworks.com/mf0/Connector/R2020b\"],\"version\":\"1.0\"}"
      mask Help: web("DocumentationPDUCDUAssemblyTL.html")
      mask DialogControl Container10 Prompt: PDU Racks
      mask DialogControl getRatingButton Prompt: Get Rating
      mask DialogControl Container5_2 Prompt: CDU
      mask DialogControl Container13 Prompt: Pumps
      mask DialogControl Container8_2 Prompt: Set External Fluid Properties
      mask DialogControl Container7_2 Prompt: Set Internal Fluid Properties
      mask DialogControl Container9_2 Prompt: Heat Transfer
      mask DialogControl Container14 Prompt: Reference Properties
      mask DialogControl Container9 Prompt: IT Tray
      mask DialogControl Container6 Prompt: GPU
      mask DialogControl Container7 Prompt: CPU
      mask DialogControl Container8 Prompt: Initial Conditions
      mask Display: image('icon_AssemblyTL.png');
  PDU + CDU Assembly (TL-TL) : Subsystem  mask{nAssembly=3, nTrays=6, nRacks=4, nPumps=1, pumpNominalRPM=3500, pumpCapacityVec=2:2:24, pumpRefHeadVec=[239, 238.5, 232, 230, 222, 216, 208, 196, 186, 170,150,130], pumpRefBrkPowVec=[0.3,0.4,0.45,0.5,0.55,0.6,0.65,0.7,0.75,0.78,0.79,0.798], pumpEff=[20,40,50,60,65,70,75,75,75,73,68,60]/100, speedLimFactor=1, pumpImpellerDiaFactor=1, extFluidMdot=[.3, .5, 1, 1.3, 1.7, 2, 2.6, 3.3], extFluidPrDrop=ones(1,8), extFluidVol=0.01, extFluidPipeArea=0.01, intFluidMdot=[.3, .5, .6, .7, 1, 1.4, 1.9, 2.3], intFluidPrDrop=ones(1,8), intFluidVol=0.01, intFluidPipeArea=0.01, spDissipationTbl=[.324, .3533, .404, .4253, .4333, .4373, .4453, .4533; .3813, .424, .496, .5307, .544, .5547, .5693, .5787; .4267, .4827, .5813, .6173, .6413, .6573, .672, .6827; .4613, .528, .64, .6987, .7267, .7467, .7707, .7853; .5533, .6467, .8227, .928, .9853, 1.0187, 1.0653, 1.0973; .58, .688, .8853, 1.0147, 1.08, 1.124, 1.176, 1.2147; .624, .7467, .992, 1.148, 1.244, 1.304, 1.3773, 1.4267; .656, .7907, 1.0667, 1.26, 1.376, 1.452, 1.548, 1.612], refT=293, refP=0.101325, refDensity=998, trayMass=5, trayCp=2000, trayThermalR=0.1, pipeLen=1, pipeArea=1e-3, pipeDia=5e-3, pipeLenXtra=0.05, thermalKtc=0.01, nGPU=1, gpuTDPperDie=1200, gpuIdlePower=300, gpuHBMpower=80, gpuExponent=1.4, gpuHBMutil=0.7, gpuLeakage=1.5, gpuNominalDieT=350, gpuDieThermalC=50, gpuHeatSinkR=0.15, gpuSurfArea=0.01, gpuAmbientR=0.5, nCPU=1, cpuTDPperSocket=350, cpuIdlePower=80, cpuExponent=1.1, cpuLeakage=1.5, cpuNominalDieT=350, cpuDieThermalC=50, cpuHeatSinkR=0.15, cpuSurfArea=0.01, cpuAmbientR=0.5, initialT=350, initialP=0.101325, htc=10}
      mask prompts: nAssembly "Number of PDU+CDU assemblies (-)"; nTrays "Number of IT trays per rack (-)"; nRacks "Number of racks (-)"; nPumps "Total number of pumps (-)"; pumpNominalRPM "Pump nominal rating (rpm)"; pumpCapacityVec "Reference capacity vector for each pump (m^3/s)"; pumpRefHeadVec "Reference head vector for each pump (m)"; pumpRefBrkPowVec "Reference brake power vector (kW)"; pumpEff "Electrical efficiency vector, 0-1 (-)"; speedLimFactor "Pump speed upper limit factor (-)"; pumpImpellerDiaFactor "Impeller diameter scale factor (-)"; extFluidMdot "External liquid loop mass flow rate vector (kg/s)"; extFluidPrDrop "External liquid loop pressure drop vector (kPa)"; extFluidVol "External liquid volume in heat exchanger (m^3)"; extFluidPipeArea "External liquid loop pipe cross-sectional area (m^2)"; intFluidMdot "Internal liquid loop mass flow rate vector (kg/s)"; intFluidPrDrop "Internal liquid loop pressure drop vector (kPa)"; intFluidVol "Internal liquid volume in heat exchanger (m^3)"; intFluidPipeArea "Internal liquid loop pipe cross-sectional area (m^2)"; spDissipationTbl "Specific dissipation table, SD[mdot_int,mdot_ext] (kW/K)"; refT "Reference flow temperature (K)"; refP "Reference flow pressure (MPa)"; refDensity "Reference density for internal liquid (kg/m^3)"; trayMass "Tray mass (kg)"; trayCp "Tray specific heat capacity (J/kg*K)"; trayThermalR "Tray to external thermal resistance (K/W)"; pipeLen "Cold plate pipe length (m)"; pipeArea "Cold plate pipe cross-sectional area (m^2)"; pipeDia "Cold plate pipe hydraulic diameter (m)"; pipeLenXtra "Cold plate pipe aggregate equivalent length of local resistances (m)"; thermalKtc "Tray to cold plate thermal resistance (K/W)"; nGPU "Number of GPU per tray (-)"; gpuTDPperDie "GPU TDP per die (W)"; gpuIdlePower "GPU idle power (W)"; gpuHBMpower "HBM power per GPU (W)"; gpuExponent "GPU power utilization exponent (-)"; gpuHBMutil "HBM utilization as fraction of compute utilization (-)"; gpuLeakage "Leakage increase per K above nominal temperature (W/K)"; gpuNominalDieT "Nominal die temperature at TDP (K)"; gpuDieThermalC "GPU die thermal capacitance (J/K)"; gpuHeatSinkR "GPU die-heat-sink thermal resistance (K/W)"; gpuSurfArea "Surface area per die for ambient heat transfer (m^2)"; gpuAmbientR "GPU die-ambient thermal resistance (K/W)"; nCPU "Number of CPU per tray (-)"; cpuTDPperSocket "CPU TDP per socket (W)"; cpuIdlePower "CPU idle power per socket (W)"; cpuExponent "CPU power utilization exponent (-)"; cpuLeakage "Leakage increase per K above nominal temperature (W/K)"; cpuNominalDieT "Nominal die temperature at TDP (K)"; cpuDieThermalC "CPU die thermal capacitance (J/K)"; cpuHeatSinkR "CPU die-heat-sink thermal resistance (K/W)"; cpuSurfArea "Surface area per die for ambient heat transfer (m^2)"; cpuAmbientR "CPU die-ambient thermal resistance (K/W)"; initialT "Initial temperature (K)"; initialP "Initial pressure (MPa)"; htc "Heat transfer coefficient to ambient (W/m^2.K)"
      settings: CopyFcn=set_param(gcbh,'LinkStatus','none');  PortSchema="{\"entries\":[{\"content\":{\"sides\":[{\"content\":{\"connectorIds\":[\"LConn1\",\"LConn2\",\"LConn3\",\"LConn4\",\"LConn5\"]},\"type\":\"ConnectorPlacement.EquallySpacedRectSide\",\"uuid\":\"c3c2deed-cbbd-4247-9ad8-92266cae4888\"},{\"content\":{\"connectorIds\":[\"RConn1\",\"RConn2\",\"RConn3\",\"RConn4\"],\"side\":\"RIGHT\"},\"type\":\"ConnectorPlacement.EquallySpacedRectSide\",\"uuid\":\"76c347ba-a09e-43ac-9cd7-77a64cbfa06b\"},{\"content\":{\"side\":\"TOP\"},\"type\":\"ConnectorPlacement.EquallySpacedRectSide\",\"uuid\":\"42a451f0-8c6e-4292-b7e5-775225f62bd3\"},{\"content\":{\"connectorIds\":[\"RConn5\",\"RConn6\"],\"side\":\"BOTTOM\"},\"type\":\"ConnectorPlacement.EquallySpacedRectSide\",\"uuid\":\"9855950e-5626-47f1-87fc-c4196e6fccba\"}]},\"type\":\"ConnectorPlacement.EquallySpacedConnector\",\"uuid\":\"03434805-a51b-483c-9948-e3fbab74b7d0\"}],\"packageUris\":[\"http://schema.mathworks.com/mf0/Connector/R2020b\"],\"version\":\"1.0\"}"
      mask Help: web("DocumentationPDUCDUAssemblyTLTL.html")
      mask DialogControl Container10 Prompt: PDU Racks
      mask DialogControl getRatingButton Prompt: Get Rating
      mask DialogControl Container5_2 Prompt: CDU
      mask DialogControl Container12 Prompt: Pump
      mask DialogControl Container8_2 Prompt: Set External Fluid Properties
      mask DialogControl Container7_2 Prompt: Set Internal Fluid Properties
      mask DialogControl Container14 Prompt: Heat Transfer
      mask DialogControl Container13 Prompt: Reference Properties
      mask DialogControl Container9 Prompt: IT Tray
      mask DialogControl Container6 Prompt: GPU
      mask DialogControl Container7 Prompt: CPU
      mask DialogControl Container8 Prompt: Initial Conditions
      mask Display: image('icon_AssemblyTLTL.png');
